simulink model "mrefrobotarm_previous_y_previous_u_previous_ref_cover_test"  (R2018b)
settings: Solver=FixedStepAuto  StartTime=0.0  StopTime=20  RelTol=1e-3  AbsTol=1e-6
undefined symbols (not defined in the file or in its folder): cc, options
libraries: neural x66, simulink x2
(part 4 of 4)

== system mrefrobotarm_previous_y_previous_u_previous_ref_cover_test/Feed-Forward Neural Network1/Layer 3/Delays 1 ==
  "p{3}" : Inport  PortDimensions=30
      mask Display: e = 0.06;c1 = [120 230 180]/255;c2 = ([120 230 180]+0)/(256+128);c3 = ([120 230 180]+128)/(256+128);patch([0 1 1 0],[0 0 1 1],c1);patch([0 1 1 1-e 1-e 0+e],[0 0 1 1-e 0+e 0+e],c2);patch([0 0 1 1-e 0+e 0+e],[0 1 1 1-e 1-e 0+e],c3);plot([0 1 1 0 0],[0 0 1 1 0]);
  mux : Mux  Inputs=1
      mask Display: e = 0.06;c1 = [120 150 230]/255;c2 = ([120 150 230]+0)/383;c3 = ([120 150 230]+128)/383;patch([0 1 1 0],[0 0 1 1],c1);patch([0 1 1 1-e 1-e 0+e],[0 0 1 1-e 0+e 0+e],c2);patch([0 0 1 1-e 0+e 0+e],[0 1 1 1-e 1-e 0+e],c3);plot([0 1 1 0 0],[0 0 1 1 0]);disp('Mux')
  "pd{3,2}" : Outport
      mask Display: e = 0.06;c1 = [120 230 180]/255;c2 = ([120 230 180]+0)/(256+128);c3 = ([120 230 180]+128)/(256+128);patch([0 1 1 0],[0 0 1 1],c1);patch([0 1 1 1-e 1-e 0+e],[0 0 1 1-e 0+e 0+e],c2);patch([0 0 1 1-e 0+e 0+e],[0 1 1 1-e 1-e 0+e],c3);plot([0 1 1 0 0],[0 0 1 1 0]);
  wires:
  "p{3}"/1 -> mux/1
  mux/1 -> "pd{3,2}"/1

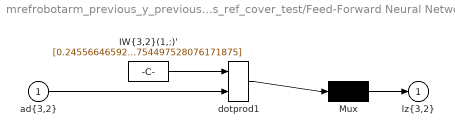
== system mrefrobotarm_previous_y_previous_u_previous_ref_cover_test/Feed-Forward Neural Network1/Layer 3/LW{3,2} ==
  "ad{3,2}" : Inport  PortDimensions=30
      mask Display: e = 0.06;c1 = [120 230 180]/255;c2 = ([120 230 180]+0)/(256+128);c3 = ([120 230 180]+128)/(256+128);patch([0 1 1 0],[0 0 1 1],c1);patch([0 1 1 1-e 1-e 0+e],[0 0 1 1-e 0+e 0+e],c2);patch([0 0 1 1-e 0+e 0+e],[0 1 1 1-e 1-e 0+e],c3);plot([0 1 1 0 0],[0 0 1 1 0]);
  "IW{3,2}(1,:)'" : Constant  Value=[0.245566465926212396109207247718586586415767669677734375;-0.56322081322037842454619749332778155803680419921875;-0.28991010367060410235495737651945091784000396728515625;0.3869683333504421174353637979947961866855621337890625;0.496517765752567064030387200546101666986942291259765625;-0.320943780837954883988771825897856615483760833740234375;0.0286370319336148211608605862465992686338722705841064453125;-0.15395906619913668489374458658858202397823333740234375;0.51493301451079076525019218024681322276592254638671875;-0.026941881639260277514491548345176852308213710784912109375;-0.05589778476223307424053388103857287205755710601806640625;0.1600136141061642980343293629630352370440959930419921875;-0.2212967731759021561277478440388222225010395050048828125;-0.168090459815553538991395043922238983213901519775390625;-0.4615503546136172641212169764912687242031097412109375;-0.60839853859597503582534727684105746448040008544921875;0.1504483327033876438605375369661487638950347900390625;-0.4073407234202310878146136019495315849781036376953125;0.331316055045982882365507293798145838081836700439453125;-0.1747391852843100945591459094430319964885711669921875;-0.19591165143500910428286942988052032887935638427734375;0.1816474984983245388736605718804639764130115509033203125;0.3783772749804861224021124144201166927814483642578125;0.046857186277910960192638611943038995377719402313232421875;-0.292883801455053660589555875048972666263580322265625;0.480373124807368323541112431485089473426342010498046875;-0.0158594532240923617727457184400918777100741863250732421875;-0.0228072195102398851684899483416302246041595935821533203125;-0.55934110245892210144802447757683694362640380859375;0.2422309302660256846717601320051471702754497528076171875]
      mask Display: e = 0.06;c1 = [120 150 230]/255;c2 = ([120 150 230]+0)/383;c3 = ([120 150 230]+128)/383;patch([0 1 1 0],[0 0 1 1],c1);patch([0 1 1 1-e 1-e 0+e],[0 0 1 1-e 0+e 0+e],c2);patch([0 0 1 1-e 0+e 0+e],[0 1 1 1-e 1-e 0+e],c3);plot([0 1 1 0 0],[0 0 1 1 0]);disp('weights');
  Mux : Mux  Inputs=1
      mask Display: e = 0.06;c1 = [120 150 230]/255;c2 = ([120 150 230]+0)/383;c3 = ([120 150 230]+128)/383;patch([0 1 1 0],[0 0 1 1],c1);patch([0 1 1 1-e 1-e 0+e],[0 0 1 1-e 0+e 0+e],c2);patch([0 0 1 1-e 0+e 0+e],[0 1 1 1-e 1-e 0+e],c3);plot([0 1 1 0 0],[0 0 1 1 0]);disp('Mux');
  dotprod1 : neural/Weight Functions/dotprod
  "lz{3,2}" : Outport
      mask Display: e = 0.06;c1 = [120 230 180]/255;c2 = ([120 230 180]+0)/(256+128);c3 = ([120 230 180]+128)/(256+128);patch([0 1 1 0],[0 0 1 1],c1);patch([0 1 1 1-e 1-e 0+e],[0 0 1 1-e 0+e 0+e],c2);patch([0 0 1 1-e 0+e 0+e],[0 1 1 1-e 1-e 0+e],c3);plot([0 1 1 0 0],[0 0 1 1 0]);
  wires:
  "IW{3,2}(1,:)'"/1 -> dotprod1/1
  "ad{3,2}"/1 -> dotprod1/2
  dotprod1/1 -> Mux/1
  Mux/1 -> "lz{3,2}"/1
